simulink library "target_generation_lib"  (R2016b)
settings: Solver=VariableStepAuto  StartTime=0.0  StopTime=10.0  RelTol=1e-3
settings Model: Creator=taylorreynolds  LastModifiedBy=Taylor

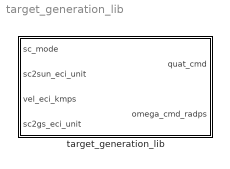
== system target_generation_lib ==
  target_generation_lib : Subsystem

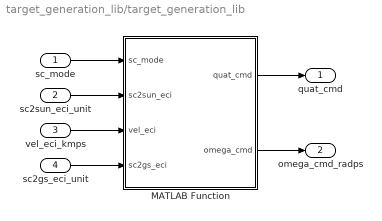
== system target_generation_lib/target_generation_lib ==
  sc_mode : Inport
  sc2sun_eci_unit : Inport  Port=2
  vel_eci_kmps : Inport  Port=3
  sc2gs_eci_unit : Inport  Port=4
  MATLAB Function : MATLAB Function  TreatAsAtomicUnit=on
  quat_cmd : Outport
  omega_cmd_radps : Outport  Port=2
  wires:
  sc_mode/1 -> MATLAB Function/1(sc_mode)
  sc2sun_eci_unit/1 -> MATLAB Function/2(sc2sun_eci)
  vel_eci_kmps/1 -> MATLAB Function/3(vel_eci)
  sc2gs_eci_unit/1 -> MATLAB Function/4(sc2gs_eci)
  MATLAB Function/1(quat_cmd) -> quat_cmd/1
  MATLAB Function/2(omega_cmd) -> omega_cmd_radps/1

== matlab function target_generation_lib/MATLAB Function ==
  data: sc_mode input; quat_cmd output; sc2sun_eci input; vel_eci input; sc2gs_eci input; omega_cmd output
function [quat_cmd,omega_cmd] = target_gen(sc_mode,sc2sun_eci,vel_eci,sc2gs_eci)
% #codegen
% FSW Target Generation Library
%   UW HuskySat-1, ADCS Team
%   Last Updated: T. Reynolds 12.27.17

% Computes desired quaternion and angular velocity depending on the sc_mode
%   mode_logic.bdot             = 1;
%   mode_logic.desat_eclipse    = 2;
%   mode_logic.point            = 3;
%       point.velocity          = 31;
%       point.ground            = 32;
%       point.MPC               = 33;
%   mode_logic.low_power        = 4;

% Body vectors of key components
COM2    = [ 0; -1; 0 ];
PPT     = [ 0; 0; -1 ];
SP      = [ 0; 1; 0 ];

% Default values in case point.MPC is active
quat_cmd    = [1; 0; 0; 0];
omega_cmd   = [0; 0; 0];

if( sc_mode == 1 || sc_mode == 2 || sc_mode == 4 )
    quat_cmd    = [1; 0; 0; 0];
    omega_cmd   = [0; 0; 0];
else
    if( sc_mode == 31 )
        r1  = vel_eci./norm(vel_eci);
        r2  = cross(r1,sc2sun_eci);
        r2  = r2./norm(r2);
        r3  = cross(r1,r2);
        b1  = -PPT;
        b2  = cross(b1,SP);
        b3  = cross(b1,b2);
        DCM_cmd     = TRIAD(r1,r2,r3,b1,b2,b3);
        quat_cmd    = my_dcm2quat(DCM_cmd);
        omega_cmd   = [0; 0; 0]; % Fill this in with mean motion
    elseif( sc_mode == 32 )
        r1  = sc2gs_eci;
        r2  = cross(r1,sc2sun_eci);
        r2  = r2./norm(r2);
        r3  = cross(r1,r2);
        b1  = [0; -1; 0];
        b2  = [sind(2); cosd(2); 0]; % rotate COM2 vector 2deg to avoid singularity issues
        b3  = [0; 0; -1];
        DCM_cmd     = TRIAD(r1,r2,r3,b1,b2,b3);
        quat_cmd    = my_dcm2quat(DCM_cmd);
        omega_cmd   = [0; 0; 0]; % Fill this in with mean motion
    end
end

end

function C = TRIAD(r1,r2,r3,b1,b2,b3)
    C   = b1*r1' + b2*r2' + b3*r3';
end

function q = my_dcm2quat( dcm )

q   = zeros(4,1);
tr  = trace(dcm);

if (tr > 0)
    sqtrp1 = sqrt( tr + 1.0 );
    
    q(1) = 0.5*sqtrp1;
    q(2) = (dcm(2, 3) - dcm(3, 2))/(2.0*sqtrp1);
    q(3) = (dcm(3, 1) - dcm(1, 3))/(2.0*sqtrp1);
    q(4) = (dcm(1, 2) - dcm(2, 1))/(2.0*sqtrp1);
else
    d = diag(dcm);
    if ((d(2) > d(1)) && (d(2) > d(3)))
        % max value at dcm(2,2,i)
        sqdip1 = sqrt(d(2) - d(1) - d(3) + 1.0 );
        
        q(3) = 0.5*sqdip1;
        
        if ( sqdip1 ~= 0 )
            sqdip1 = 0.5/sqdip1;
        end
        
        q(1) = (dcm(3, 1) - dcm(1, 3))*sqdip1;
        q(2) = (dcm(1, 2) + dcm(2, 1))*sqdip1;
        q(4) = (dcm(2, 3) + dcm(3, 2))*sqdip1;
    elseif (d(3) > d(1))
        % max value at dcm(3,3,i)
        sqdip1 = sqrt(d(3) - d(1) - d(2) + 1.0 );
        
        q(4) = 0.5*sqdip1;
        
        if ( sqdip1 ~= 0 )
            sqdip1 = 0.5/sqdip1;
        end
        
        q(1) = (dcm(1, 2) - dcm(2, 1))*sqdip1;
        q(2) = (dcm(3, 1) + dcm(1, 3))*sqdip1;
        q(3) = (dcm(2, 3) + dcm(3, 2))*sqdip1;
    else
        % max value at dcm(1,1,i)
        sqdip1 = sqrt(d(1) - d(2) - d(3) + 1.0 );
        
        q(2) = 0.5*sqdip1;
        
        if ( sqdip1 ~= 0 )
            sqdip1 = 0.5/sqdip1;
        end
        
        q(1) = (dcm(2, 3) - dcm(3, 2))*sqdip1;
        q(3) = (dcm(1, 2) + dcm(2, 1))*sqdip1;
        q(4) = (dcm(3, 1) + dcm(1, 3))*sqdip1;
    end
end

end
